simulink model "hil0_host_demo"  (Simulink 7.3)
settings: Solver=ode3  StartTime=0.0  StopTime=5  FixedStep=0.005  RelTol=1e-3
settings Model: Creator=Krisada  LastModifiedBy=Krisada

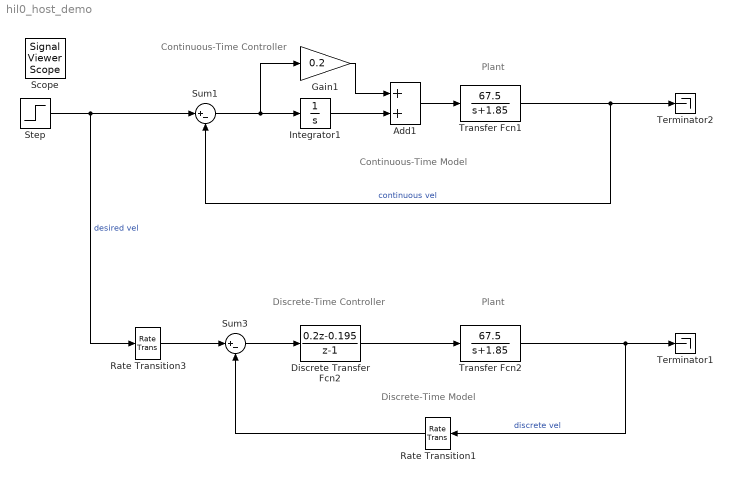
== system hil0_host_demo ==
  note: Discrete-Time Model
  note: Continuous-Time Model
  note: Plant
  note: Continuous-Time Controller
  note: Discrete-Time Controller
  note: Plant
  Add1 : Sum  OutDataType=fixdt(1, 16)  OutScaling=2^-10
  Discrete Transfer Fcn2 : DiscreteTransferFcn  Numerator=[0.2 -0.195]  Denominator=[1 -1]  SampleTime=-1
  Gain1 : Gain  Gain=0.2  ParameterDataType=fixdt(1, 16)  ParameterScaling=2^0  OutDataType=fixdt(1, 16)  OutScaling=2^0
  Integrator1 : Integrator
  Rate Transition1 : RateTransition  OutPortSampleTime=0.005
  Rate Transition3 : RateTransition  OutPortSampleTime=0.005
  Step : Step  After=700  SampleTime=0
  Sum1 : Sum  Inputs=|+-  OutDataType=fixdt(1, 16)  OutScaling=2^0
  Sum3 : Sum  Inputs=|+-  OutDataType=fixdt(1, 16)  OutScaling=2^0
  Terminator1 : Terminator
  Terminator2 : Terminator
  Transfer Fcn1 : TransferFcn  Numerator=67.5  Denominator=[1 1.85]
  Transfer Fcn2 : TransferFcn  Numerator=67.5  Denominator=[1 1.85]
  Scope : SignalViewerScope  IOType=viewer  LegendLocations="371.3333      357.6667           127      51.66667"  RefreshTime=0.035000
      settings: ShowLegends=on  YMin=0  YMax=800
  wires:
  Step/1 -> Sum1/1, Rate Transition3/1  "desired vel"
  Rate Transition3/1 -> Sum3/1
  Transfer Fcn2/1 -> Terminator1/1, Rate Transition1/1  "discrete vel"
  Sum3/1 -> Discrete Transfer Fcn2/1
  Discrete Transfer Fcn2/1 -> Transfer Fcn2/1
  Rate Transition1/1 -> Sum3/2
  Transfer Fcn1/1 -> Terminator2/1, Sum1/2  "continuous vel"
  Sum1/1 -> Gain1/1, Integrator1/1
  Integrator1/1 -> Add1/2
  Gain1/1 -> Add1/1
  Add1/1 -> Transfer Fcn1/1
